simulink model "ofdm2011"  (Simulink 7.1)
settings: Solver=ode45  StartTime=0.0  StopTime=0.08  RelTol=1e-3
undefined symbols (not defined in the file): Fs, get, rsgenpoly
libraries: dspobslib x9, commdigbbndpm2 x6, dspbuff3 x4, dspstat3 x4, commsink2 x4, dspindex x4, dspsrcs4 x2, dspxfrm3 x2, commblkcod2 x2, commseqgen2 x2, commutil2 x2, commchan3 x1
Description:
  | This COFDM Simulation simulate Coded OFDM using
  | Reed-Solomon Channel Coding, over wireless multipath
  | fading channel, with 3 us maximal delay spread, 200 Hz
  | Doppler shift.
  | In this simulation I use QPSK, and Training Based
  | Channel Estimation, 11/15 RS Code, 2 Symbol Error
  | Correction
  | 
  | I also have paper that report this simulation in
  | Matlab Central
  | 
  | If you interest about this simulation, please mail to
  | gito_pras@telkom.net
settings Model: Creator=Gito Prastomo  LastModifiedBy=wen
settings SolverCC: MaxConsecutiveZCs=10
settings DataIOCC: SignalLoggingName=sigsOut
settings DebuggingCC: SaveWithParameterizedLinksMsg=none  SignalResolutionControl=TryResolveAllWithWarning  SolverPrmCheckMsg=none  MultiTaskDSMMsg=warning  MultiTaskCondExecSysMsg=none  StrictBusMsg=None
settings HardwareCC: TargetUnknown=on
settings RTWCC: IncludeERTFirstTime=on

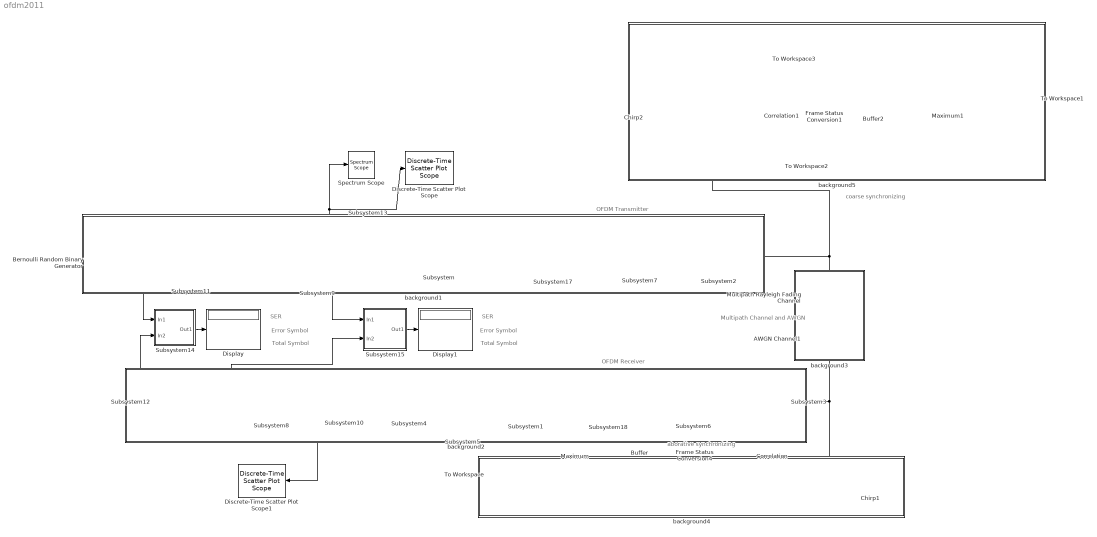
== system ofdm2011 ==
  note: SER
  note: Error Symbol
  note: Total Symbol
  note: SER
  note: Error Symbol
  note: Total Symbol
  note: OFDM Receiver
  note: OFDM Transmitter
  note: Multipath Channel
      | and AWGN
  note: aborative synchronizing
  note: coarse synchronizing
  AWGN Channel1 : commchan3/AWGN Channel  Orientation=down  SystemSampleTime=-1  seed=32965  noiseMode="Signal to noise ratio  (SNR)"  EbNodB=10  EsNodB=28  SNRdB=10  bitsPerSym=1  Ps=30/(5.5e5*11/15*2.4)*1.08  Tsym=80e-6  variance=1
  Bernoulli Random Binary Generator : commrandsrc2/Bernoulli Binary Generator  DialogController=commDDGCreate  DialogControllerArgs=DataTag0  SystemSampleTime=-1  P=[0.5]  seed=9364248  Ts=16e-5/44/2  frameBased=on  sampPerFrame=44  orient=off  outDataType=double
  Buffer : dspbuff3/Buffer  Orientation=left  N=180  V=0  ic=0
  Buffer2 : dspbuff3/Buffer  N=180  V=0  ic=0
  Chirp1 : dspsrcs4/Chirp  Orientation=left  sweep=Linear  mode=Unidirectional  f0=6000  f1=9000  t1=0.01  Tsweep=1  phase=0  Ts=1/1000  spf=1  datatype=Double
  Chirp2 : dspsrcs4/Chirp  sweep=Linear  mode=Unidirectional  f0=6000  f1=9000  t1=0.01  Tsweep=1  phase=0  Ts=1/1000  spf=1  datatype=Double
  Correlation : dspstat3/Correlation  Orientation=left  DialogController=dspDDGCreate  DialogControllerArgs=DataTag1  domain=Time  roundingMode=Floor  overflowMode=off
  Correlation1 : dspstat3/Correlation  DialogController=dspDDGCreate  DialogControllerArgs=DataTag2  domain=Time  roundingMode=Floor  overflowMode=off
  Discrete-Time Scatter Plot Scope : commsink2/Discrete-Time Scatter Plot Scope  Tag=ScatterPlot  SystemSampleTime=-1  sampPerSymb=1  offsetEye=0  numTraces=40  numNewFrames=10  LineMarkers=.  LineColors=b  fading=on  render=on  AxisGrid=on  xMin=-3.3  xMax=3.315  yMin=-3.3  yMax=3.315  inphaseLabel=In-phase Amplitude  quadratureLabel=Quadrature Amplitude  openScopeAtSimStart=on  FrameNumber=off  FigPos=get(0,'defaultfigureposition');  figTitle=Scatter Plot  numLinesMax=8  block_type_=scatter
  Discrete-Time Scatter Plot Scope1 : commsink2/Discrete-Time Scatter Plot Scope  Tag=ScatterPlot  Orientation=left  SystemSampleTime=-1  sampPerSymb=1  offsetEye=0  numTraces=40  numNewFrames=10  LineMarkers=.  LineColors=b  fading=on  render=on  AxisGrid=on  xMin=-3.3  xMax=3.315  yMin=-3.3  yMax=3.315  inphaseLabel=In-phase Amplitude  quadratureLabel=Quadrature Amplitude  openScopeAtSimStart=on  FrameNumber=off  FigPos=get(0,'defaultfigureposition');  figTitle=Scatter Plot  numLinesMax=8  block_type_=scatter
  Display : Display
  Display1 : Display
  Frame Status Conversion1 : dspobslib/Frame Status Conversion  SystemSampleTime=-1  growRefPort=off  outframe=Frame-based
  Frame Status Conversion4 : dspobslib/Frame Status Conversion  Orientation=left  SystemSampleTime=-1  growRefPort=off  outframe=Frame-based
  Maximum : dspstat3/Maximum  Orientation=left  DialogController=dspfixptddg.MinMax  DialogControllerArgs=DataTag3  fcn=Index  reset=None  indexBase=One  operateOver=Each column  Dimension=1  colComp=on  operation=maximum  roundingMode=Floor  overflowMode=off
  Maximum1 : dspstat3/Maximum  DialogController=dspfixptddg.MinMax  DialogControllerArgs=DataTag4  fcn=Index  reset=None  indexBase=One  operateOver=Each column  Dimension=1  colComp=on  operation=maximum  roundingMode=Floor  overflowMode=off
  Multipath Rayleigh Fading Channel : commchan2/Multipath Rayleigh Fading Channel  Orientation=down  SystemSampleTime=-1  Fd=200  simTs=8e-5/180  delayVec=[0 3e-6]  gainVecdB=[0 -40]  normGain=on  Seed=936497248
  Spectrum Scope : dspsnks4/Spectrum Scope  DialogController=dspdialog.SpectrumScope  DialogControllerArgs=DataTag5  SystemSampleTime=-1  ScopeProperties=off  Domain=Frequency  HorizSpan=1  UseBuffer=on  BufferSize=1024  Overlap=512  inpFftLenInherit=on  FFTlength=1024  numAvg=64  DisplayProperties=off  AxisGrid=on  Memory=off  FrameNumber=on  AxisLegend=off  AxisZoom=off  OpenScopeAtSimStart=on  OpenScopeImmediately=off  FigPos=get(0,'defaultfigureposition')  AxisProperties=on  XUnits=Hertz  XRange=[-Fs/2...Fs/2]  XDisplay=0  InheritXIncr=on  XIncr=1.0  XLabel=Samples  XLimit=Auto  YUnits=dB  XMax=1  XMin=0  YLabel=Magnitude, dB  LineProperties=off  wintypeSpecScope=Hann  RsSpecScope=50  betaSpecScope=5  winsampSpecScope=Periodic
      settings: YMin=-30  YMax=15
  Subsystem : Subsystem
      mask Display: disp('OFDM Baseband\nModulator\ndan\nAdd Cyclic Prefix')
  Subsystem1 : Subsystem  Orientation=left
      mask Display: disp('OFDM Baseband\nDemodulator\ndan \nRemove Cyclic prefix')
  Subsystem10 : Subsystem  Orientation=left
      mask Display: disp('Remove\nZero')
  Subsystem11 : Subsystem
      mask Display: disp('RS(15,11) Encoder')
  Subsystem12 : Subsystem  Orientation=left
      mask Display: disp('RS(15,11) Decoder')
  Subsystem13 : Subsystem
      mask Display: disp('Training')
  Subsystem14 : Subsystem
      mask Display: disp('SER\nCalculation')
  Subsystem15 : Subsystem
      mask Display: disp('SER\nCalculation')
  Subsystem17 : Subsystem
      mask Display: disp('Add\nCyclic Prefix')
  Subsystem18 : Subsystem  Orientation=left
      mask Display: disp('Remove\nCyclic Prefix')
  Subsystem2 : Subsystem
      mask Display: disp('P/S')
  Subsystem3 : Subsystem  Orientation=left
      mask Display: disp('S/P')
  Subsystem4 : Subsystem  Orientation=left
      mask Display: disp('Channel\nCompensation')
  Subsystem5 : Subsystem  Orientation=left
      mask Display: disp('Channel\nEstimator')
  Subsystem6 : Subsystem  Orientation=left
      mask Display: disp('Training\nSeparation')
  Subsystem7 : Subsystem
      mask Display: disp('Training\nInsertion')
  Subsystem8 : Subsystem  Orientation=left
      mask Display: disp('QPSK Demapping')
  Subsystem9 : Subsystem
      mask Display: disp('QPSK Mapping')
  To Workspace : ToWorkspace  VariableName=xcorr_max  SampleTime=-1  SaveFormat=Array
  To Workspace1 : ToWorkspace  VariableName=xcorr_max1  SampleTime=-1  SaveFormat=Array
  To Workspace2 : ToWorkspace  VariableName=chirp  SampleTime=-1  SaveFormat=Array
  To Workspace3 : ToWorkspace  VariableName=DATA_receive  SampleTime=-1  SaveFormat=Array
  background1 : Subsystem
      mask Display: disp('')
  background2 : Subsystem
      mask Display: disp('')
  background3 : Subsystem
      mask Display: disp('')
  background4 : Subsystem
      mask Display: disp('')
  background5 : Subsystem
      mask Display: disp('')
  wires:
  Bernoulli Random Binary Generator/1 -> Subsystem11/1(In1), Subsystem14/1(In1)
  Subsystem11/1(Out1) -> Subsystem9/1(In1), Subsystem15/1(In1)
  Subsystem9/1(Out1) -> Subsystem/2(In2), Discrete-Time Scatter Plot Scope/1, Spectrum Scope/1
  Subsystem13/1(Out1) -> Subsystem/1(In1)
  Subsystem12/1(Out1) -> Subsystem14/2(In2)
  Subsystem8/1(Out1) -> Subsystem12/1(In1), Subsystem15/2(In2)
  Subsystem/1(Out1) -> Subsystem17/1(In1)
  Subsystem7/1(Out1) -> Subsystem2/1(In1)
  Subsystem6/1(Out1) -> Subsystem18/1(In1)
  Subsystem14/1(Out1) -> Display/1
  Subsystem3/1(Out1) -> Subsystem6/1(In1)
  Subsystem2/1(Out1) -> Multipath Rayleigh Fading Channel/1, To Workspace3/1, Correlation1/1
  Subsystem10/1(Out1) -> Subsystem8/1(In1), Discrete-Time Scatter Plot Scope1/1
  Multipath Rayleigh Fading Channel/1 -> AWGN Channel1/1
  AWGN Channel1/1 -> Subsystem3/1(In1), Correlation/1
  Subsystem15/1(Out1) -> Display1/1
  Subsystem4/1(Out1) -> Subsystem10/1(In1)
  Subsystem1/1(Out1) -> Subsystem4/1(In1)
  Subsystem5/1(Out1) -> Subsystem4/2(In2)
  Subsystem1/2(Out2) -> Subsystem5/1(In1)
  Subsystem17/1(Out1) -> Subsystem7/1(In1)
  Subsystem18/1(Out1) -> Subsystem1/1(In1)
  Buffer/1 -> Maximum/1
  Correlation/1 -> Frame Status Conversion4/1
  Chirp1/1 -> Correlation/2
  Frame Status Conversion4/1 -> Buffer/1
  Maximum/1 -> To Workspace/1
  Correlation1/1 -> Frame Status Conversion1/1
  Maximum1/1 -> To Workspace1/1
  Chirp2/1 -> To Workspace2/1, Correlation1/2
  Buffer2/1 -> Maximum1/1
  Frame Status Conversion1/1 -> Buffer2/1

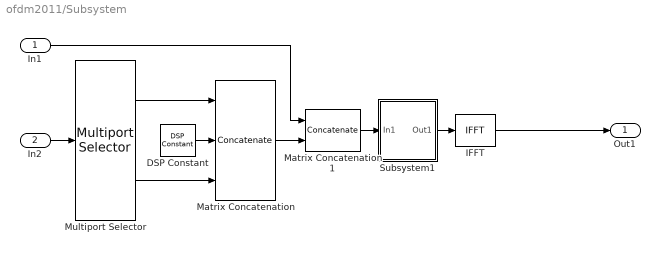
== system ofdm2011/Subsystem ==
  In1 : Inport  OutDataType=sfix(16)  OutScaling=2^0
  In2 : Inport  Port=2  OutDataType=sfix(16)  OutScaling=2^0
  DSP Constant : dspobslib/DSP Constant  SystemSampleTime=-1  Value=0  SampleMode=Discrete  discreteOutput=Frame-based  continuousOutput=Sample-based  sampTime=16e-5/2  framePeriod=16e-5/2  dataType=Inherit from 'Constant value'  isSigned=on  wordLen=16  udDataType=sfix(16)  fracBitsMode=Best precision  numFracBits=15  InterpretAs1D=off  Ts=16e-5/2  FramebasedOutput=on
  IFFT : dspxfrm3/IFFT  DialogController=dspDDGCreate  DialogControllerArgs=DataTag6  CompMethod=Table lookup  TableOpt=Speed  BitRevOrder=off  cs_in=off  SkipNorm=off  InheritFFTLength=on  FFTLength=64  mode=Real  roundingMode=Floor  overflowMode=off
  Matrix Concatenation : Concatenate  NumInputs=3  Mode=Multidimensional array
  Matrix Concatenation1 : Concatenate  Mode=Multidimensional array  ConcatenateDimension=2
  Multiport Selector : dspindex/Multiport Selector  rowsOrCols=Rows  idxCellArray={1:15,16:30}  idxErrMode=Clip Index
  Subsystem1 : Subsystem
      mask Display: disp('Zero Pad')
  Out1 : Outport
  wires:
  IFFT/1 -> Out1/1
  Multiport Selector/1 -> Matrix Concatenation/1
  Multiport Selector/2 -> Matrix Concatenation/3
  DSP Constant/1 -> Matrix Concatenation/2
  Subsystem1/1(Out1) -> IFFT/1
  In2/1 -> Multiport Selector/1
  Matrix Concatenation1/1 -> Subsystem1/1(In1)
  Matrix Concatenation/1 -> Matrix Concatenation1/2
  In1/1 -> Matrix Concatenation1/1

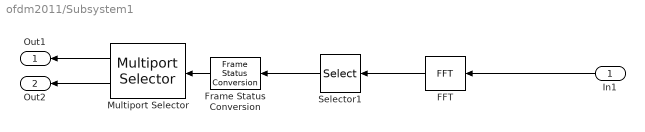
== system ofdm2011/Subsystem1 ==
  In1 : Inport  Orientation=left  OutDataType=sfix(16)  OutScaling=2^0
  FFT : dspxfrm3/FFT  Orientation=left  DialogController=dspDDGCreate  DialogControllerArgs=DataTag7  CompMethod=Table lookup  TableOpt=Speed  BitRevOrder=off  InheritFFTLength=on  FFTLength=64  SkipNorm=on  roundingMode=Floor  overflowMode=off
  Frame Status Conversion : dspobslib/Frame Status Conversion  Orientation=left  SystemSampleTime=-1  growRefPort=off  outframe=Frame-based
  Multiport Selector : dspindex/Multiport Selector  Orientation=left  rowsOrCols=Columns  idxCellArray={1,2}  idxErrMode=Clip Index
  Selector1 : Selector  Orientation=left  NumberOfDimensions=2  InputPortWidth=64  IndexOptions=Index vector (dialog),Select all  Indices=[50:64,1:16],-1  OutputSizes=1
  Out1 : Outport  Orientation=left
  Out2 : Outport  Orientation=left  Port=2
  wires:
  FFT/1 -> Selector1/1
  Selector1/1 -> Frame Status Conversion/1
  In1/1 -> FFT/1
  Frame Status Conversion/1 -> Multiport Selector/1
  Multiport Selector/1 -> Out1/1
  Multiport Selector/2 -> Out2/1

== system ofdm2011/Subsystem10 ==
  In1 : Inport  Orientation=left  OutDataType=sfix(16)  OutScaling=2^0
  Selector2 : Selector  Orientation=left  NumberOfDimensions=2  InputPortWidth=31  IndexOptions=Index vector (dialog),Select all  Indices=[1:15,17:31],-1  OutputSizes=1
  Out1 : Outport  Orientation=left
  wires:
  Selector2/1 -> Out1/1
  In1/1 -> Selector2/1

== system ofdm2011/Subsystem11 ==
  In1 : Inport  OutDataType=sfix(16)  OutScaling=2^0
  Binary-Input RS Encoder : commblkcod2/Binary-Input RS Encoder  SystemSampleTime=-1  n=15  k=11  specPrimPoly=off  primPoly=[1 0 1 1]  specGenPoly=off  genPoly=rsgenpoly(7,3)  specPuncture=off  punctVec=[ones(2,1); zeros(2,1)]  outDType=Same as input
  Out1 : Outport
  wires:
  In1/1 -> Binary-Input RS Encoder/1
  Binary-Input RS Encoder/1 -> Out1/1

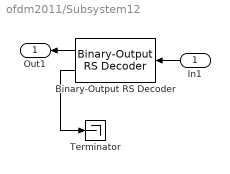
== system ofdm2011/Subsystem12 ==
  In1 : Inport  Orientation=left  OutDataType=sfix(16)  OutScaling=2^0
  Binary-Output RS Decoder : commblkcod2/Binary-Output RS Decoder  Orientation=left  SystemSampleTime=-1  n=15  k=11  specPrimPoly=off  primPoly=[1 0 1 1]  specGenPoly=off  genPoly=rsgenpoly(7,3)  specPuncture=off  punctVec=[ones(2,1); zeros(2,1)]  specErasurePort=off  showNumErr=on  outDType=Same as input
  Terminator : Terminator
  Out1 : Outport  Orientation=left
  wires:
  Binary-Output RS Decoder/2 -> Terminator/1
  Binary-Output RS Decoder/1 -> Out1/1
  In1/1 -> Binary-Output RS Decoder/1

== system ofdm2011/Subsystem13 ==
  PN Sequence Generator : commseqgen2/PN Sequence Generator  poly=[1 0 0 0 0 1 1]  ini_sta=[0 0 0 0 0 1]  outBitMaskSource=Dialog parameter  shift=0  Ts=16e-5/2/31  frameBased=on  sampPerFrame=31  reset=off  bitPackedOutputs=off  outDataType=double  numPackedBits=8  bitPackDataSigned=off  bitPackedOutDType=double
  Unipolar to Bipolar Converter : commutil2/Unipolar to Bipolar Converter  SystemSampleTime=-1  M=2  polarity=Positive  dataType=Inherit via internal rule
  Out1 : Outport
  wires:
  PN Sequence Generator/1 -> Unipolar to Bipolar Converter/1
  Unipolar to Bipolar Converter/1 -> Out1/1

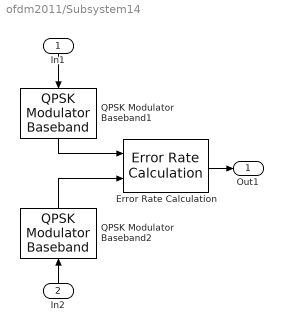
== system ofdm2011/Subsystem14 ==
  In1 : Inport  Orientation=down  OutDataType=sfix(16)  OutScaling=2^0
  In2 : Inport  Orientation=up  Port=2  OutDataType=sfix(16)  OutScaling=2^0
  Error Rate Calculation : commsink2/Error Rate Calculation  N=22  st_delay=0  cp_mode=Entire frame  subframe=[]  PMode=Port  WsName=ErrorVec  RsMode2=off  stop=off  numErr=inf  maxBits=2e4
  QPSK Modulator Baseband1 : commdigbbndpm2/QPSK Modulator Baseband  Orientation=down  SystemSampleTime=-1  InType=Bit  Enc=Gray  Ph=pi/4  numSamp=1
  QPSK Modulator Baseband2 : commdigbbndpm2/QPSK Modulator Baseband  Orientation=up  SystemSampleTime=-1  InType=Bit  Enc=Gray  Ph=pi/4  numSamp=1
  Out1 : Outport
  wires:
  QPSK Modulator Baseband1/1 -> Error Rate Calculation/1
  QPSK Modulator Baseband2/1 -> Error Rate Calculation/2
  In1/1 -> QPSK Modulator Baseband1/1
  Error Rate Calculation/1 -> Out1/1
  In2/1 -> QPSK Modulator Baseband2/1

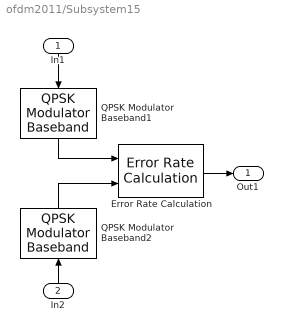
== system ofdm2011/Subsystem15 ==
  In1 : Inport  Orientation=down  OutDataType=sfix(16)  OutScaling=2^0
  In2 : Inport  Orientation=up  Port=2  OutDataType=sfix(16)  OutScaling=2^0
  Error Rate Calculation : commsink2/Error Rate Calculation  N=30  st_delay=0  cp_mode=Entire frame  subframe=[]  PMode=Port  WsName=ErrorVec  RsMode2=off  stop=off  numErr=inf  maxBits=2e4
  QPSK Modulator Baseband1 : commdigbbndpm2/QPSK Modulator Baseband  Orientation=down  SystemSampleTime=-1  InType=Bit  Enc=Gray  Ph=pi/4  numSamp=1
  QPSK Modulator Baseband2 : commdigbbndpm2/QPSK Modulator Baseband  Orientation=up  SystemSampleTime=-1  InType=Bit  Enc=Gray  Ph=pi/4  numSamp=1
  Out1 : Outport
  wires:
  QPSK Modulator Baseband1/1 -> Error Rate Calculation/1
  QPSK Modulator Baseband2/1 -> Error Rate Calculation/2
  In1/1 -> QPSK Modulator Baseband1/1
  Error Rate Calculation/1 -> Out1/1
  In2/1 -> QPSK Modulator Baseband2/1

== system ofdm2011/Subsystem17 ==
  In1 : Inport  OutDataType=sfix(16)  OutScaling=2^0
  Selector3 : Selector  NumberOfDimensions=2  InputPortWidth=64  IndexOptions=Index vector (dialog),Select all  Indices=[39:64,1:64],-1  OutputSizes=1
  Out1 : Outport
  wires:
  Selector3/1 -> Out1/1
  In1/1 -> Selector3/1

== system ofdm2011/Subsystem18 ==
  In1 : Inport  Orientation=left  OutDataType=sfix(16)  OutScaling=2^0
  Selector4 : Selector  Orientation=left  NumberOfDimensions=2  InputPortWidth=78  IndexOptions=Index vector (dialog),Select all  Indices=[27:90],-1  OutputSizes=1
  Out1 : Outport  Orientation=left
  wires:
  Selector4/1 -> Out1/1
  In1/1 -> Selector4/1

== system ofdm2011/Subsystem2 ==
  In1 : Inport  OutDataType=sfix(16)  OutScaling=2^0
  Unbuffer3 : dspbuff3/Unbuffer  ic=0
  Out1 : Outport
  wires:
  In1/1 -> Unbuffer3/1
  Unbuffer3/1 -> Out1/1

== system ofdm2011/Subsystem3 ==
  In1 : Inport  Orientation=left  OutDataType=sfix(16)  OutScaling=2^0
  Buffer : dspbuff3/Buffer  Orientation=left  N=180  V=0  ic=0
  Out1 : Outport  Orientation=left
  wires:
  In1/1 -> Buffer/1
  Buffer/1 -> Out1/1

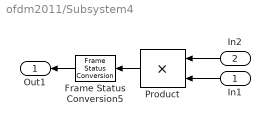
== system ofdm2011/Subsystem4 ==
  In1 : Inport  Orientation=left  OutDataType=sfix(16)  OutScaling=2^0
  In2 : Inport  Orientation=left  Port=2  OutDataType=sfix(16)  OutScaling=2^0
  Frame Status Conversion5 : dspobslib/Frame Status Conversion  Orientation=left  SystemSampleTime=-1  growRefPort=off  outframe=Frame-based
  Product : Product  Orientation=left  OutDataType=sfix(16)  OutScaling=2^0  SaturateOnIntegerOverflow=on  OutDataTypeStr=Inherit: Same as first input
  Out1 : Outport  Orientation=left
  wires:
  Frame Status Conversion5/1 -> Out1/1
  In2/1 -> Product/1
  Product/1 -> Frame Status Conversion5/1
  In1/1 -> Product/2

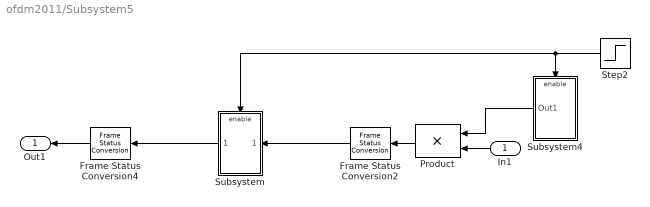
== system ofdm2011/Subsystem5 ==
  In1 : Inport  Orientation=left  OutDataType=sfix(16)  OutScaling=2^0
  Frame Status Conversion2 : dspobslib/Frame Status Conversion  Orientation=left  SystemSampleTime=-1  growRefPort=off  outframe=Frame-based
  Frame Status Conversion4 : dspobslib/Frame Status Conversion  Orientation=left  SystemSampleTime=-1  growRefPort=off  outframe=Frame-based
  Product : Product  Orientation=left  OutDataType=sfix(16)  OutScaling=2^0  SaturateOnIntegerOverflow=on  OutDataTypeStr=Inherit: Same as first input
  Step2 : Step  Orientation=left  Time=16e-5/2  SampleTime=16e-5/2
  Subsystem : Subsystem  Orientation=left
  Subsystem4 : Subsystem  Orientation=left  TreatAsAtomicUnit=on
  Out1 : Outport  Orientation=left
  wires:
  Step2/1 -> Subsystem4/Enable, Subsystem/Enable
  Subsystem4/1(Out1) -> Product/1
  Product/1 -> Frame Status Conversion2/1
  Frame Status Conversion2/1 -> Subsystem/1(In1)
  Frame Status Conversion4/1 -> Out1/1
  In1/1 -> Product/2
  Subsystem/1(Out1) -> Frame Status Conversion4/1

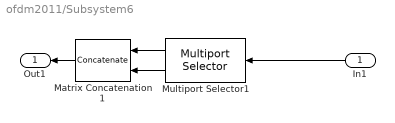
== system ofdm2011/Subsystem6 ==
  In1 : Inport  Orientation=left  OutDataType=sfix(16)  OutScaling=2^0
  Matrix Concatenation1 : Concatenate  Orientation=left  Mode=Multidimensional array  ConcatenateDimension=2
  Multiport Selector1 : dspindex/Multiport Selector  Orientation=left  rowsOrCols=Rows  idxCellArray={91:180,1:90}  idxErrMode=Clip Index
  Out1 : Outport  Orientation=left
  wires:
  Multiport Selector1/2 -> Matrix Concatenation1/2
  Multiport Selector1/1 -> Matrix Concatenation1/1
  In1/1 -> Multiport Selector1/1
  Matrix Concatenation1/1 -> Out1/1

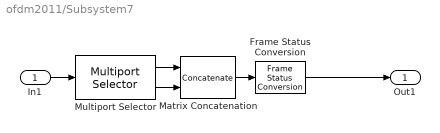
== system ofdm2011/Subsystem7 ==
  In1 : Inport  OutDataType=sfix(16)  OutScaling=2^0
  Frame Status Conversion : dspobslib/Frame Status Conversion  SystemSampleTime=-1  growRefPort=off  outframe=Frame-based
  Matrix Concatenation : Concatenate  Mode=Multidimensional array
  Multiport Selector : dspindex/Multiport Selector  rowsOrCols=Columns  idxCellArray={1,2}  idxErrMode=Clip Index
  Out1 : Outport
  wires:
  Multiport Selector/1 -> Matrix Concatenation/1
  Multiport Selector/2 -> Matrix Concatenation/2
  Matrix Concatenation/1 -> Frame Status Conversion/1
  In1/1 -> Multiport Selector/1
  Frame Status Conversion/1 -> Out1/1

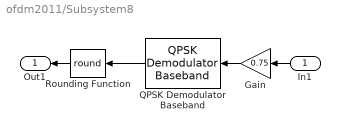
== system ofdm2011/Subsystem8 ==
  In1 : Inport  Orientation=left  OutDataType=sfix(16)  OutScaling=2^0
  Gain : Gain  Orientation=left  Gain=0.75  ParameterDataType=sfix(16)  ParameterScaling=2^0  OutDataType=sfix(16)  OutScaling=2^0  SaturateOnIntegerOverflow=on  OutDataTypeStr=Inherit: Same as input  ParamDataTypeStr=Inherit: Same as input
  QPSK Demodulator Baseband : commdigbbndpm2/QPSK Demodulator Baseband  Orientation=left  SystemSampleTime=-1  OutType=Bit  Dec=Gray  Ph=pi/4  numSamp=1
  Rounding Function : Rounding  Orientation=left  Operator=round
  Out1 : Outport  Orientation=left
  wires:
  In1/1 -> Gain/1
  Rounding Function/1 -> Out1/1
  QPSK Demodulator Baseband/1 -> Rounding Function/1
  Gain/1 -> QPSK Demodulator Baseband/1

== system ofdm2011/Subsystem9 ==
  In1 : Inport  OutDataType=sfix(16)  OutScaling=2^0
  Gain : Gain  Gain=1/0.75  ParameterDataType=sfix(16)  ParameterScaling=2^0  OutDataType=sfix(16)  OutScaling=2^0  SaturateOnIntegerOverflow=on  OutDataTypeStr=Inherit: Same as input  ParamDataTypeStr=Inherit: Same as input
  QPSK Modulator Baseband : commdigbbndpm2/QPSK Modulator Baseband  SystemSampleTime=-1  InType=Bit  Enc=Gray  Ph=pi/4  numSamp=1
  Out1 : Outport
  wires:
  QPSK Modulator Baseband/1 -> Gain/1
  In1/1 -> QPSK Modulator Baseband/1
  Gain/1 -> Out1/1

== system ofdm2011/background1 ==

== system ofdm2011/background2 ==

== system ofdm2011/background3 ==

== system ofdm2011/background4 ==

== system ofdm2011/background5 ==

== system ofdm2011/Subsystem/Subsystem1 ==
  In1 : Inport  OutDataType=sfix(16)  OutScaling=2^0
  Selector : Selector  NumberOfDimensions=2  InputPortWidth=64  IndexOptions=Index vector (dialog),Select all  Indices=[16:64,1:15],-1  OutputSizes=1
  Zero Pad : dspsigops/Pad  padAlong=Columns and rows  dimsToPad=1  valSrc=Specify via dialog  padVal=0  spec=Output size  padNumOutRowsSpecMethod=User-specified  numOutRows=64  padNumOutColsSpecMethod=User-specified  numOutCols=2  isVarDimsMode=off  padBeginning=0  padEnd=0  outSizeMode=User-specified  outSize=1  padSigAt=End  trunc_flag=None  roundingMode=Floor  overflowMode=off  truncOrWrapMode=Truncate  wrap_flag=None
  Out1 : Outport
  wires:
  Zero Pad/1 -> Selector/1
  In1/1 -> Zero Pad/1
  Selector/1 -> Out1/1

== system ofdm2011/Subsystem5/Subsystem ==
  In1 : Inport  Orientation=left  OutDataType=sfix(16)  OutScaling=2^0
  Enable : EnablePort
  Math Function : Math  Orientation=left  Operator=reciprocal  SaturateOnIntegerOverflow=on
  Out1 : Outport  Orientation=left
  wires:
  In1/1 -> Math Function/1
  Math Function/1 -> Out1/1

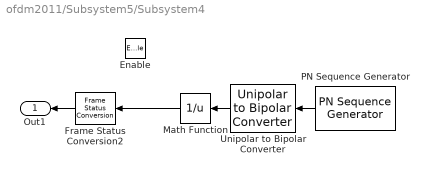
== system ofdm2011/Subsystem5/Subsystem4 ==
  Enable : EnablePort
  Frame Status Conversion2 : dspobslib/Frame Status Conversion  Orientation=left  SystemSampleTime=-1  growRefPort=off  outframe=Frame-based
  Math Function : Math  Orientation=left  Operator=reciprocal  SaturateOnIntegerOverflow=on
  PN Sequence Generator : commseqgen2/PN Sequence Generator  Orientation=left  poly=[1 0 0 0 0 1 1]  ini_sta=[0 0 0 0 0 1]  outBitMaskSource=Dialog parameter  shift=0  Ts=16e-5/2/31  frameBased=on  sampPerFrame=31  reset=off  bitPackedOutputs=off  outDataType=double  numPackedBits=8  bitPackDataSigned=off  bitPackedOutDType=double
  Unipolar to Bipolar Converter : commutil2/Unipolar to Bipolar Converter  Orientation=left  SystemSampleTime=-1  M=2  polarity=Positive  dataType=Inherit via internal rule
  Out1 : Outport  Orientation=left
  wires:
  PN Sequence Generator/1 -> Unipolar to Bipolar Converter/1
  Frame Status Conversion2/1 -> Out1/1
  Math Function/1 -> Frame Status Conversion2/1
  Unipolar to Bipolar Converter/1 -> Math Function/1
